simulink model "Task"  (R2018b)
settings: Solver=FixedStepDiscrete  StartTime=0.0  StopTime=10.0  RelTol=1e-3
settings Model: Creator=Mostafa  LastModifiedBy=Mostafa
settings ConfigSet: Description=Mostafa Hany Imam
settings OptimizationCC: DefaultParameterBehavior=Inlined  EnhancedBackFolding=on  PassReuseOutputArgsAs=Individual arguments  OptimizeBlockOrder=speed  DifferentSizesBufferReuse=on  OptimizationCustomize=off
settings DebuggingCC: UnderspecifiedInitializationDetection=Classic  MergeDetectMultiDrivingBlocksExec=none  ParameterTunabilityLossMsg=error
settings ModelReferenceCC: PropagateSignalLabelsOutOfModel=off
settings SFSimCC: MATLABDynamicMemAlloc=off
settings RTWCC: SystemTargetFile=ert.tlc  GenCodeOnly=on  TemplateMakefile=ert_default_tmf  GenerateReport=on  IncludeHyperlinkInReport=on  LaunchReport=on  GenerateTraceInfo=on  GenerateTraceReport=on  GenerateTraceReportSl=on  GenerateTraceReportSf=on  GenerateTraceReportEml=on
settings CodeAppCC: ForceParamTrailComments=on  IgnoreCustomStorageClasses=off  OperatorAnnotations=on  SimulinkDataObjDesc=on  SFDataObjDesc=on  InsertBlockDesc=on
settings ERTTargetCC: TargetLangStandard=C99 (ISO)  GenerateSampleERTMain=on  InlinedParameterPlacement=NonHierarchical  ERTCustomFileTemplate=example_file_process.tlc

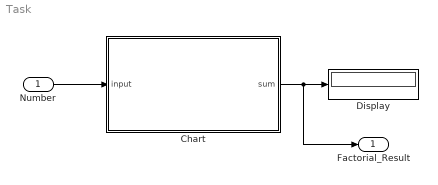
== system Task ==
  Number : Inport
  Chart : Stateflow chart  TreatAsAtomicUnit=on
  Display : Display
  "Factorial_Result " : Outport
  wires:
  Number/1 -> Chart/1(input)
  Chart/1(sum) -> "Factorial_Result "/1, Display/1

== stateflow chart Task/Chart ==
  (default) -> (junction 12) : /* Factorial */
  (junction 13) -> (junction 11) [order 1] : [index <=input]
  (junction 11) -> (junction 14) : {sum = sum * index;}
  (junction 12) -> (junction 13) : {index = 1;sum = 1;}
  (junction 14) -> (junction 13) : {index=index+1;}
  (junction 13) -> (junction 15) [order 2]
  data: index local uint32; sum output uint32; input input uint32
